simulink library "mylib"  (R2020b)
settings: Solver=VariableStepAuto  StartTime=0.0  StopTime=10.0  RelTol=1e-3
libraries: powerlib x4
settings Model: Creator=janluca  LastModifiedBy=janluca

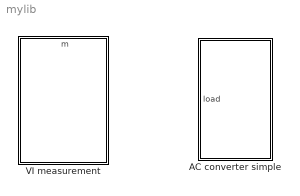
== system mylib ==
  AC converter simple : Subsystem  mask{eff=1}
      mask prompts: eff "Efficiency"
  VI measurement : Subsystem
      settings: PortSchema="{\"entries\":[{\"content\":{\"sides\":[{\"content\":{\"connectorIds\":[\"LConn1\",\"LConn2\"]},\"type\":\"ConnectorPlacement.EquallySpacedRectSide\",\"uuid\":\"f3b73344-d0cf-4b93-ad96-f780fa5a1256\"},{\"content\":{\"connectorIds\":[\"RConn1\",\"RConn2\"],\"side\":\"RIGHT\"},\"type\":\"ConnectorPlacement.EquallySpacedRectSide\",\"uuid\":\"030ebb8c-daa3-4185-a78c-b002204e2a62\"},{\"content\":{\"connectorIds\":[\"Out1\"],\"side\":\"TOP\"},\"type\":\"ConnectorPlacement.EquallySpacedRectSide\",\"uuid\":\"0cc05069-4c24-40a7-976e-8b87ed915541\"},{\"content\":{\"connectorIds\":[],\"side\":\"HIDDEN\"},\"type\":\"ConnectorPlacement.EquallySpacedRectSide\",\"uuid\":\"da030f82-010e-483f-97d7-c36c3edfce40\"}]},\"type\":\"ConnectorPlacement.EquallySpacedConnector\",\"uuid\":\"1bb0f634-fa5d-4f47-8259-a0e02a201bbc\"}],\"packageUris\":[\"http://schema.mathworks.com/mf0/Connector/R2020b\"],\"version\":\"1.0\"}"

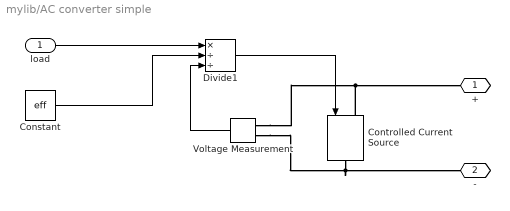
== system mylib/AC converter simple ==
  load : Inport
  Constant : Constant  Value=eff
  Controlled Current Source : powerlib/Electrical Sources/Controlled Current Source  Initialize=on  Source_Type=AC  Amplitude=0  Phase=0  Frequency=0  Measurements=None
  Divide1 : Product  Inputs=*//
  Voltage Measurement : powerlib/Measurements/Voltage Measurement  PhasorSimulation=off  OutputType=Complex  PSBequivalent=0
  + : PMIOPort  Side=Right
  - : PMIOPort  Port=2  Side=Right
  wires:
  load/1 -> Divide1/1
  Divide1/1 -> Controlled Current Source/1
  Constant/1 -> Divide1/2
  Voltage Measurement/1 -> Divide1/3
  connections:
  Controlled Current Source/RConn1 -- Voltage Measurement/LConn2 -- -/RConn1
  Controlled Current Source/LConn1 -- Voltage Measurement/LConn1 -- +/RConn1

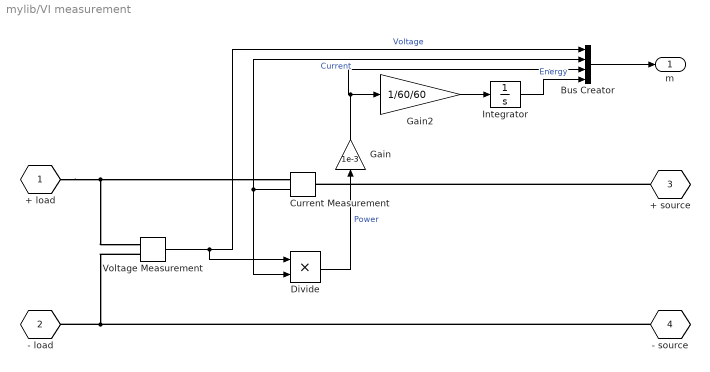
== system mylib/VI measurement ==
  Bus Creator : BusCreator  Inputs=4
  Current Measurement : powerlib/Measurements/Current Measurement  PhasorSimulation=off  OutputType=Complex  PSBequivalent=0
  Divide : Product  Inputs=**
  Gain : Gain  Gain=1e-3
  Gain2 : Gain  Gain=1/60/60
  Integrator : Integrator
  Voltage Measurement : powerlib/Measurements/Voltage Measurement  PhasorSimulation=off  OutputType=Complex  PSBequivalent=0
  + load : PMIOPort  Tag=PMCPort  Side=Left
  - load : PMIOPort  Tag=PMCPort  Port=2  Side=Left
  + source : PMIOPort  Tag=PMCPort  Port=3  Side=Right
  - source : PMIOPort  Tag=PMCPort  Port=4  Side=Right
  m : Outport
  wires:
  Voltage Measurement/1 -> Divide/1, Bus Creator/1  "Voltage"
  Current Measurement/1 -> Bus Creator/2, Divide/2  "Current"
  Divide/1 -> Gain/1  "Power"
  Bus Creator/1 -> m/1
  Gain2/1 -> Integrator/1
  Integrator/1 -> Bus Creator/4  "Energy"
  Gain/1 -> Bus Creator/3, Gain2/1
  connections:
  + load/RConn1 -- Current Measurement/RConn1 -- Voltage Measurement/LConn1
  Voltage Measurement/LConn2 -- - load/RConn1 -- - source/RConn1
  + source/RConn1 -- Current Measurement/LConn1
